simulink model "gm_DUALportRAMinterface_v3_vnl"  (R2024a)
settings: Solver=FixedStepDiscrete  StartTime=0.0  StopTime=20  RelTol=1e-3
undefined symbols (not defined in the file or in its folder): magnitude, Ts
libraries: hdlsllib x419, hdlmdlgenlib x103, embmathops x12, simulink x5, dsphdlxfrm2 x2
(part 4 of 11)

== system gm_DUALportRAMinterface_v3_vnl/PL/integration_block1/GA_main/Chart ==
  sort_done : Inport  OutDataTypeStr=boolean  PortDimensions=1  SampleTime=3.00000003e-08
  start_GA : Inport  Port=2  OutDataTypeStr=boolean  PortDimensions=1  SampleTime=3.00000003e-08
  score_done : Inport  Port=3  OutDataTypeStr=boolean  PortDimensions=1  SampleTime=3.00000003e-08
  FIFO_full : Inport  Port=4  OutDataTypeStr=boolean  PortDimensions=1  SampleTime=3.00000003e-08
  random_gene : Inport  Port=5  OutDataTypeStr=fixdt(0, 3, 0)  PortDimensions=1  SampleTime=3.00000003e-08
  selected_method : Inport  Port=6  OutDataTypeStr=fixdt(0, 3, 0)  PortDimensions=1  SampleTime=3.00000003e-08
  sample_index : Inport  Port=7  OutDataTypeStr=fixdt(0, 4, 0)  PortDimensions=1  SampleTime=3.00000003e-08
  generation_counter : Inport  Port=8  OutDataTypeStr=uint16  PortDimensions=1  SampleTime=3.00000003e-08
  Chart : Stateflow chart  TreatAsAtomicUnit=on
      settings: PortSchema="{\"entries\":[{\"content\":{\"sides\":[{\"content\":{\"connectorIds\":[\"In1\",\"In2\",\"In3\",\"In4\",\"In5\",\"In6\",\"In7\",\"In8\"]},\"type\":\"ConnectorPlacement.EquallySpacedRectSide\",\"uuid\":\"62d80992-ebbf-487b-a33b-520d46b16df9\"},{\"content\":{\"connectorIds\":[\"Out1\",\"Out4\",\"Out5\",\"Out6\",\"Out8\",\"Out9\",\"Out7\",\"Out10\",\"Out11\",\"Out12\",\"Out15\",\"Out16\",\"Out13\",\"Out14\",\"Out3\",\"Out2\",\"Out17\",\"Out18\"],\"side\":\"RIGHT\"},\"type\":\"ConnectorPlacement.EquallySpacedRectSide\",\"uuid\":\"bfd840c0-5c4c-4a80-a2e3-fe311b40edf5\"},{\"content\":{\"side\":\"TOP\"},\"type\":\"ConnectorPlacement.EquallySpacedRectSide\",\"uuid\":\"4ac6e66e-dbf9-46cb-9f74-339923e0521f\"},{\"content\":{\"side\":\"BOTTOM\"},\"type\":\"ConnectorPlacement.EquallySpacedRectSide\",\"uuid\":\"c9defcd3-49e4-4e79-8497-0d4d1ccc3a89\"}]},\"type\":\"ConnectorPlacement.EquallySpacedConnector\",\"uuid\":\"f0f6ce29-0824-409a-b95e-7d534cdcf216\"}],\"packageUris\":[\"http://schema.mathworks.com/mf0/Connector/R2020b\"],\"version\":\"1.0\"}"
  GA_done : Outport  SampleTime=3.00000003e-08
  index_reset : Outport  Port=2  SampleTime=3.00000003e-08
  index_increment : Outport  Port=3  SampleTime=3.00000003e-08
  a2_method : Outport  Port=4  SampleTime=3.00000003e-08
  a3_method : Outport  Port=5  SampleTime=3.00000003e-08
  a4_method : Outport  Port=6  SampleTime=3.00000003e-08
  b4_method : Outport  Port=7  SampleTime=3.00000003e-08
  b2_method : Outport  Port=8  SampleTime=3.00000003e-08
  b3_method : Outport  Port=9  SampleTime=3.00000003e-08
  slave_input : Outport  Port=10  SampleTime=3.00000003e-08
  slave_output : Outport  Port=11  SampleTime=3.00000003e-08
  master_input : Outport  Port=12  SampleTime=3.00000003e-08
  generation_increment : Outport  Port=13  SampleTime=3.00000003e-08
  generation_reset : Outport  Port=14  SampleTime=3.00000003e-08
  master_output : Outport  Port=15  SampleTime=3.00000003e-08
  master_sort : Outport  Port=16  SampleTime=3.00000003e-08
  FIFO_out_en : Outport  Port=17  SampleTime=3.00000003e-08
  load_fifo : Outport  Port=18  SampleTime=3.00000003e-08
  wires:
  Chart/18(load_fifo) -> load_fifo/1
  Chart/17(FIFO_out_en) -> FIFO_out_en/1
  Chart/16(master_sort) -> master_sort/1
  Chart/15(master_output) -> master_output/1
  Chart/14(generation_reset) -> generation_reset/1
  Chart/13(generation_increment) -> generation_increment/1
  Chart/12(master_input) -> master_input/1
  Chart/11(slave_output) -> slave_output/1
  Chart/10(slave_input) -> slave_input/1
  Chart/9(b3_method) -> b3_method/1
  Chart/8(b2_method) -> b2_method/1
  Chart/7(b4_method) -> b4_method/1
  Chart/6(a4_method) -> a4_method/1
  Chart/5(a3_method) -> a3_method/1
  Chart/4(a2_method) -> a2_method/1
  Chart/3(index_increment) -> index_increment/1
  Chart/2(index_reset) -> index_reset/1
  Chart/1(GA_done) -> GA_done/1
  generation_counter/1 -> Chart/8(generation_counter)
  sample_index/1 -> Chart/7(sample_index)
  selected_method/1 -> Chart/6(selected_method)
  random_gene/1 -> Chart/5(random_gene)
  FIFO_full/1 -> Chart/4(FIFO_full)
  score_done/1 -> Chart/3(score_done)
  start_GA/1 -> Chart/2(start_GA)
  sort_done/1 -> Chart/1(sort_done)

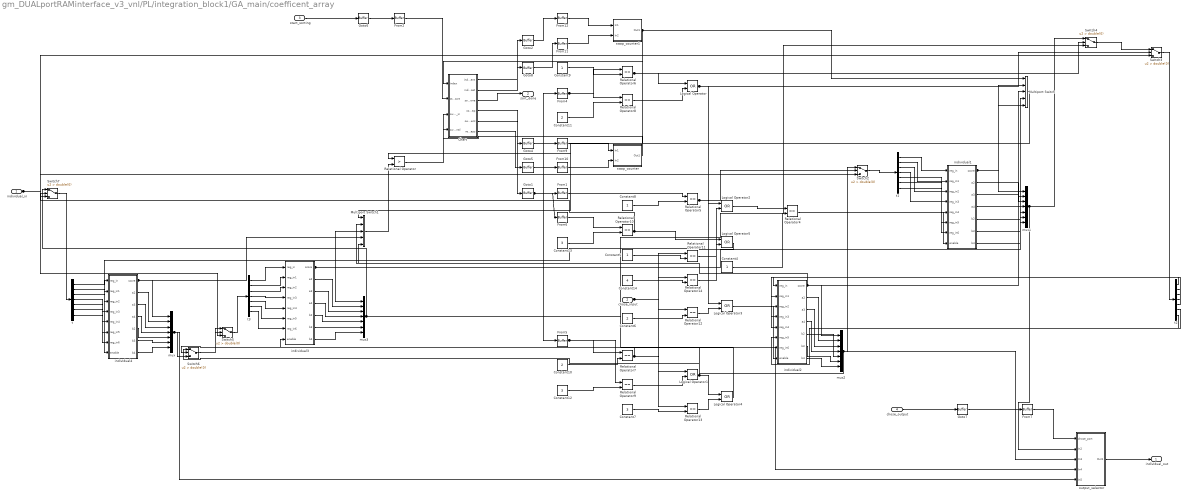
== system gm_DUALportRAMinterface_v3_vnl/PL/integration_block1/GA_main/coefficent_array ==
  individual_in : Inport  OutDataTypeStr=fixdt(1, 33, 15)  PortDimensions=[7]  SampleTime=3.00000003e-08
  chose_input : Inport  Port=2  OutDataTypeStr=fixdt(0, 4, 0)  PortDimensions=1  SampleTime=3.00000003e-08
  start_sorting : Inport  Port=3  OutDataTypeStr=boolean  PortDimensions=1  SampleTime=3.00000003e-08
  chose_output : Inport  Port=4  OutDataTypeStr=fixdt(0, 4, 0)  PortDimensions=1  SampleTime=3.00000003e-08
  Chart : Subsystem
  Constant10 : Constant  Value=2  OutDataTypeStr=fixdt(0, 4, 0)  SampleTime=3.00000003e-08
  Constant11 : Constant  Value=2  OutDataTypeStr=fixdt(0, 4, 0)  SampleTime=3.00000003e-08
  Constant12 : Constant  Value=3  OutDataTypeStr=fixdt(0, 4, 0)  SampleTime=3.00000003e-08
  Constant13 : Constant  Value=3  OutDataTypeStr=fixdt(0, 4, 0)  SampleTime=3.00000003e-08
  Constant14 : Constant  Value=4  OutDataTypeStr=fixdt(0, 4, 0)  SampleTime=3.00000003e-08
  Constant{4..5,8..9} (4 alike) : Constant  OutDataTypeStr=fixdt(0, 4, 0)  SampleTime=3.00000003e-08
  Constant6 : Constant  Value=2  OutDataTypeStr=fixdt(0, 4, 0)  SampleTime=3.00000003e-08
  Constant7 : Constant  Value=3  OutDataTypeStr=fixdt(0, 4, 0)  SampleTime=3.00000003e-08
  From{1..2,4..7,9..12} (10 alike) : hdlmdlgenlib/Buffer
  Goto{1..2,4..8} (7 alike) : hdlmdlgenlib/Buffer
  Logical Operator{,1..5} (6 alike) : Logic  Operator=OR  AllPortsSameDT=off  OutDataTypeStr=boolean  SampleTime=3.00000003e-08
  Multiport Switch : MultiPortSwitch  DataPortForDefault=Additional data port  DiagnosticForDefault=None  OutDataTypeStr=fixdt(1, 33, 15)  SampleTime=3.00000003e-08  SaturateOnIntegerOverflow=off  InputSameDT=off
  Multiport Switch1 : MultiPortSwitch  DataPortForDefault=Additional data port  DiagnosticForDefault=None  OutDataTypeStr=fixdt(1, 33, 15)  SampleTime=3.00000003e-08  SaturateOnIntegerOverflow=off  InputSameDT=off
  Relational Operator : RelationalOperator  Operator=>  OutDataTypeStr=boolean  SampleTime=3.00000003e-08  InputSameDT=off
  Relational Operator{4..14} (11 alike) : RelationalOperator  Operator===  OutDataTypeStr=boolean  SampleTime=3.00000003e-08  InputSameDT=off
  Switch{2..7} (6 alike) : Switch  Criteria=u2 > Threshold  Threshold=double(0)  OutDataTypeStr=fixdt(1, 33, 15)  SampleTime=3.00000003e-08  SaturateOnIntegerOverflow=off  InputSameDT=off
  individual1 : Subsystem
  individual2 : Subsystem
  individual3 : Subsystem
  individual4 : Subsystem
  mux{,1..3} (4 alike) : Mux  Inputs=7
  output_selector : Subsystem
  swap_counter : Subsystem
  swap_counter1 : Subsystem
  t{,1..3} (4 alike) : Demux  Outputs=7
  individual_out : Outport  SampleTime=3.00000003e-08
  sort_done : Outport  Port=2  SampleTime=3.00000003e-08
  wires:
  Switch5/1 -> t3/1
  Switch6/1 -> Switch5/1
  Switch3/1 -> t2/1
  Switch4/1 -> Switch3/1
  Switch2/1 -> t1/1
  Relational Operator5/1 -> Logical Operator2/1, Switch2/2
  From1/1 -> Relational Operator5/1
  Goto1/1 -> From1/1, From4/1, From5/1, From6/1
  Chart/6(reset_swaps) -> Goto5/1
  Chart/5(swaps_increment) -> Goto4/1
  Chart/4(commit_swap) -> Goto1/1
  Chart/2(index_reset) -> Goto8/1
  Chart/1(index_increment) -> Goto2/1
  Goto2/1 -> From12/1
  Goto8/1 -> From11/1
  Goto4/1 -> From9/1
  Goto5/1 -> From10/1
  Relational Operator/1 -> Chart/4(swap_signal)
  Multiport Switch/1 -> Relational Operator/1
  Multiport Switch1/1 -> Relational Operator/2
  Switch7/1 -> t/1
  Relational Operator10/1 -> Logical Operator5/1, Switch7/2
  From6/1 -> Relational Operator10/1
  Logical Operator2/1 -> Relational Operator4/1
  Relational Operator6/1 -> Logical Operator/1, Switch4/2
  From4/1 -> Relational Operator6/1, Relational Operator8/1
  Logical Operator/1 -> Logical Operator3/1, Switch3/2
  Relational Operator8/1 -> Logical Operator/2
  Relational Operator7/1 -> Logical Operator1/1, Switch6/2
  From5/1 -> Relational Operator7/1, Relational Operator9/1
  Logical Operator1/1 -> Logical Operator4/1, Switch5/2
  Relational Operator9/1 -> Logical Operator1/2
  t3/7 -> individual3/7(reg_in6)
  t3/6 -> individual3/6(reg_in5)
  t3/5 -> individual3/5(reg_in4)
  t3/4 -> individual3/4(reg_in3)
  t3/3 -> individual3/3(reg_in2)
  t3/2 -> individual3/2(reg_in1)
  t3/1 -> individual3/1(reg_in)
  t2/7 -> individual2/7(reg_in6)
  t2/6 -> individual2/6(reg_in5)
  t2/5 -> individual2/5(reg_in4)
  t2/4 -> individual2/4(reg_in3)
  t2/3 -> individual2/3(reg_in2)
  t2/2 -> individual2/2(reg_in1)
  t2/1 -> individual2/1(reg_in)
  t1/7 -> individual1/7(reg_in6)
  t1/6 -> individual1/6(reg_in5)
  t1/5 -> individual1/5(reg_in4)
  t1/4 -> individual1/4(reg_in3)
  t1/3 -> individual1/3(reg_in2)
  t1/2 -> individual1/2(reg_in1)
  t1/1 -> individual1/1(reg_in)
  From12/1 -> swap_counter1/1(In1)
  From11/1 -> swap_counter1/2(In2)
  From9/1 -> swap_counter/1(In1)
  From10/1 -> swap_counter/2(In2)
  t/7 -> individual4/7(reg_in6)
  t/6 -> individual4/6(reg_in5)
  t/5 -> individual4/5(reg_in4)
  t/4 -> individual4/4(reg_in3)
  t/3 -> individual4/3(reg_in2)
  t/2 -> individual4/2(reg_in1)
  t/1 -> individual4/1(reg_in)
  Logical Operator5/1 -> individual4/8(enable)
  Relational Operator4/1 -> individual1/8(enable)
  Logical Operator3/1 -> individual2/8(enable)
  Logical Operator4/1 -> individual3/8(enable)
  Constant8/1 -> Relational Operator5/2
  From2/1 -> Chart/2(start_sort)
  individual_in/1 -> Switch2/3, Switch3/3, Switch5/3, Switch7/3
  Constant13/1 -> Relational Operator10/2
  Relational Operator14/1 -> Logical Operator5/2
  Constant4/1 -> Relational Operator4/2
  Relational Operator11/1 -> Logical Operator2/2
  Constant9/1 -> Relational Operator6/2
  Constant11/1 -> Relational Operator8/2
  Relational Operator12/1 -> Logical Operator3/2
  Constant10/1 -> Relational Operator7/2
  Constant12/1 -> Relational Operator9/2
  Relational Operator13/1 -> Logical Operator4/2
  swap_counter1/1(Out1) -> Multiport Switch1/1, Multiport Switch/1, Chart/1(index)
  swap_counter/1(Out1) -> Chart/3(swaps_in)
  individual4/7(b4) -> mux/7
  individual4/6(b3) -> mux/6
  individual4/5(b2) -> mux/5
  individual4/4(a4) -> mux/4
  individual4/3(a3) -> mux/3
  individual4/2(a2) -> mux/2
  individual4/1(score) -> mux/1, Multiport Switch1/4
  individual1/7(b4) -> mux1/7
  individual1/6(b3) -> mux1/6
  individual1/5(b2) -> mux1/5
  individual1/4(a4) -> mux1/4
  individual1/3(a3) -> mux1/3
  individual1/2(a2) -> mux1/2
  individual1/1(score) -> mux1/1, Multiport Switch/5, Multiport Switch/2
  individual2/7(b4) -> mux2/7
  individual2/6(b3) -> mux2/6
  individual2/5(b2) -> mux2/5
  individual2/4(a4) -> mux2/4
  individual2/3(a3) -> mux2/3
  individual2/2(a2) -> mux2/2
  individual2/1(score) -> mux2/1, Multiport Switch1/5, Multiport Switch1/2, Multiport Switch/3
  individual3/7(b4) -> mux3/7
  individual3/6(b3) -> mux3/6
  individual3/5(b2) -> mux3/5
  individual3/4(a4) -> mux3/4
  individual3/3(a3) -> mux3/3
  individual3/2(a2) -> mux3/2
  individual3/1(score) -> mux3/1, Multiport Switch1/3, Multiport Switch/4
  Goto7/1 -> From7/1
  Goto6/1 -> From2/1
  output_selector/1(Out1) -> individual_out/1
  mux/1 -> Switch6/3, output_selector/5(In5)
  mux3/1 -> Switch4/3, Switch7/1, output_selector/4(In4)
  mux2/1 -> Switch2/1, Switch6/1, output_selector/3(In3)
  mux1/1 -> Switch4/1, output_selector/2(In2)
  From7/1 -> output_selector/1(chose_port)
  Constant7/1 -> Relational Operator13/2
  Constant6/1 -> Relational Operator12/2
  Constant5/1 -> Relational Operator11/2
  Constant14/1 -> Relational Operator14/2
  Chart/3(sort_done) -> sort_done/1
  chose_output/1 -> Goto7/1
  start_sorting/1 -> Goto6/1
  chose_input/1 -> Relational Operator11/1, Relational Operator12/1, Relational Operator13/1, Relational Operator14/1

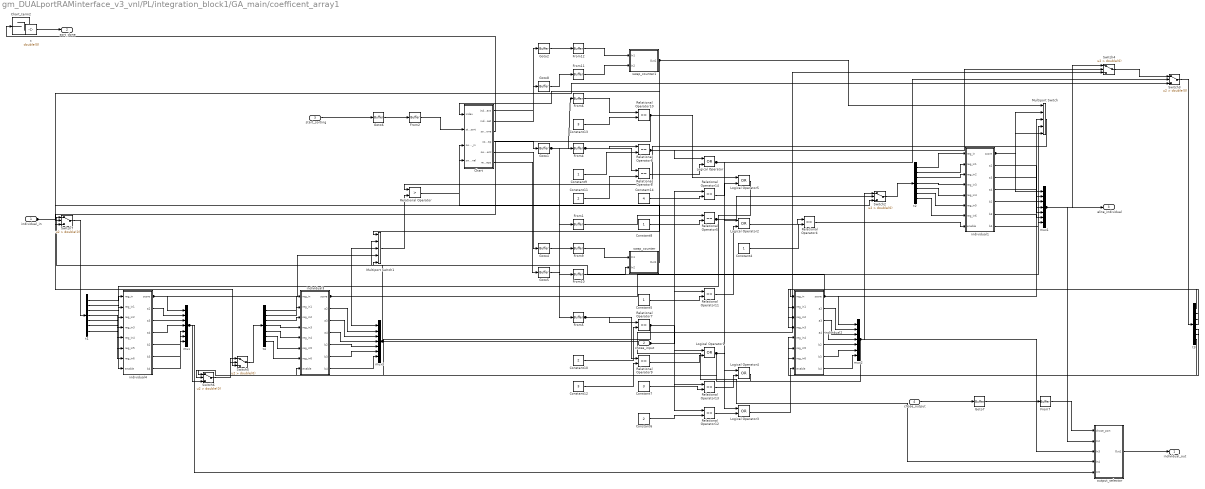
== system gm_DUALportRAMinterface_v3_vnl/PL/integration_block1/GA_main/coefficent_array1 ==
  individual_in : Inport  OutDataTypeStr=fixdt(1, 33, 15)  PortDimensions=[7]  SampleTime=3.00000003e-08
  chose_input : Inport  Port=2  OutDataTypeStr=fixdt(0, 4, 0)  PortDimensions=1  SampleTime=3.00000003e-08
  start_sorting : Inport  Port=3  OutDataTypeStr=boolean  PortDimensions=1  SampleTime=3.00000003e-08
  chose_output : Inport  Port=4  OutDataTypeStr=fixdt(0, 4, 0)  PortDimensions=1  SampleTime=3.00000003e-08
  Chart : Subsystem
  Chart_term2 : Terminator
  Constant10 : Constant  Value=2  OutDataTypeStr=fixdt(0, 4, 0)  SampleTime=3.00000003e-08
  Constant11 : Constant  Value=2  OutDataTypeStr=fixdt(0, 4, 0)  SampleTime=3.00000003e-08
  Constant12 : Constant  Value=3  OutDataTypeStr=fixdt(0, 4, 0)  SampleTime=3.00000003e-08
  Constant13 : Constant  Value=3  OutDataTypeStr=fixdt(0, 4, 0)  SampleTime=3.00000003e-08
  Constant14 : Constant  Value=4  OutDataTypeStr=fixdt(0, 4, 0)  SampleTime=3.00000003e-08
  Constant{4..5,8..9} (4 alike) : Constant  OutDataTypeStr=fixdt(0, 4, 0)  SampleTime=3.00000003e-08
  Constant6 : Constant  Value=2  OutDataTypeStr=fixdt(0, 4, 0)  SampleTime=3.00000003e-08
  Constant7 : Constant  Value=3  OutDataTypeStr=fixdt(0, 4, 0)  SampleTime=3.00000003e-08
  From{1..2,4..7,9..12} (10 alike) : hdlmdlgenlib/Buffer
  Goto{1..2,4..8} (7 alike) : hdlmdlgenlib/Buffer
  Logical Operator{,1..5} (6 alike) : Logic  Operator=OR  AllPortsSameDT=off  OutDataTypeStr=boolean  SampleTime=3.00000003e-08
  Multiport Switch : MultiPortSwitch  DataPortForDefault=Additional data port  DiagnosticForDefault=None  OutDataTypeStr=fixdt(1, 33, 15)  SampleTime=3.00000003e-08  SaturateOnIntegerOverflow=off  InputSameDT=off
  Multiport Switch1 : MultiPortSwitch  DataPortForDefault=Additional data port  DiagnosticForDefault=None  OutDataTypeStr=fixdt(1, 33, 15)  SampleTime=3.00000003e-08  SaturateOnIntegerOverflow=off  InputSameDT=off
  Relational Operator : RelationalOperator  Operator=>  OutDataTypeStr=boolean  SampleTime=3.00000003e-08  InputSameDT=off
  Relational Operator{4..14} (11 alike) : RelationalOperator  Operator===  OutDataTypeStr=boolean  SampleTime=3.00000003e-08  InputSameDT=off
  Switch{2..7} (6 alike) : Switch  Criteria=u2 > Threshold  Threshold=double(0)  OutDataTypeStr=fixdt(1, 33, 15)  SampleTime=3.00000003e-08  SaturateOnIntegerOverflow=off  InputSameDT=off
  individual1 : Subsystem
  individual2 : Subsystem
  individual3 : Subsystem
  individual4 : Subsystem
  mux{,1..3} (4 alike) : Mux  Inputs=7
  output_selector : Subsystem
  swap_counter : Subsystem
  swap_counter1 : Subsystem
  t : Constant  Value=double(0)  OutDataTypeStr=boolean  SampleTime=3.00000003e-08
  t{1..4} (4 alike) : Demux  Outputs=7
  individual_out : Outport  SampleTime=3.00000003e-08
  sort_done : Outport  Port=2  SampleTime=3.00000003e-08
  elite_individual : Outport  Port=3  SampleTime=3.00000003e-08
  wires:
  Switch5/1 -> t4/1
  Switch6/1 -> Switch5/1
  Switch3/1 -> t3/1
  Switch4/1 -> Switch3/1
  Switch2/1 -> t2/1
  Relational Operator5/1 -> Logical Operator2/1, Switch2/2
  From1/1 -> Relational Operator5/1
  Goto1/1 -> From1/1, From4/1, From5/1, From6/1
  Chart/6(reset_swaps) -> Goto5/1
  Chart/5(swaps_increment) -> Goto4/1
  Chart/4(commit_swap) -> Goto1/1
  Chart/2(index_reset) -> Goto8/1
  Chart/1(index_increment) -> Goto2/1
  Goto2/1 -> From12/1
  Goto8/1 -> From11/1
  Goto4/1 -> From9/1
  Goto5/1 -> From10/1
  Relational Operator/1 -> Chart/4(swap_signal)
  Multiport Switch/1 -> Relational Operator/1
  Multiport Switch1/1 -> Relational Operator/2
  Switch7/1 -> t1/1
  Relational Operator10/1 -> Logical Operator5/1, Switch7/2
  From6/1 -> Relational Operator10/1
  Logical Operator2/1 -> Relational Operator4/1
  Relational Operator6/1 -> Logical Operator/1, Switch4/2
  From4/1 -> Relational Operator6/1, Relational Operator8/1
  Logical Operator/1 -> Logical Operator3/1, Switch3/2
  Relational Operator8/1 -> Logical Operator/2
  Relational Operator7/1 -> Logical Operator1/1, Switch6/2
  From5/1 -> Relational Operator7/1, Relational Operator9/1
  Logical Operator1/1 -> Logical Operator4/1, Switch5/2
  Relational Operator9/1 -> Logical Operator1/2
  t4/7 -> individual3/7(reg_in6)
  t4/6 -> individual3/6(reg_in5)
  t4/5 -> individual3/5(reg_in4)
  t4/4 -> individual3/4(reg_in3)
  t4/3 -> individual3/3(reg_in2)
  t4/2 -> individual3/2(reg_in1)
  t4/1 -> individual3/1(reg_in)
  t3/7 -> individual2/7(reg_in6)
  t3/6 -> individual2/6(reg_in5)
  t3/5 -> individual2/5(reg_in4)
  t3/4 -> individual2/4(reg_in3)
  t3/3 -> individual2/3(reg_in2)
  t3/2 -> individual2/2(reg_in1)
  t3/1 -> individual2/1(reg_in)
  t2/7 -> individual1/7(reg_in6)
  t2/6 -> individual1/6(reg_in5)
  t2/5 -> individual1/5(reg_in4)
  t2/4 -> individual1/4(reg_in3)
  t2/3 -> individual1/3(reg_in2)
  t2/2 -> individual1/2(reg_in1)
  t2/1 -> individual1/1(reg_in)
  From12/1 -> swap_counter1/1(In1)
  From11/1 -> swap_counter1/2(In2)
  From9/1 -> swap_counter/1(In1)
  From10/1 -> swap_counter/2(In2)
  t1/7 -> individual4/7(reg_in6)
  t1/6 -> individual4/6(reg_in5)
  t1/5 -> individual4/5(reg_in4)
  t1/4 -> individual4/4(reg_in3)
  t1/3 -> individual4/3(reg_in2)
  t1/2 -> individual4/2(reg_in1)
  t1/1 -> individual4/1(reg_in)
  Logical Operator5/1 -> individual4/8(enable)
  Relational Operator4/1 -> individual1/8(enable)
  Logical Operator3/1 -> individual2/8(enable)
  Logical Operator4/1 -> individual3/8(enable)
  Constant8/1 -> Relational Operator5/2
  From2/1 -> Chart/2(start_sort)
  individual_in/1 -> Switch2/3, Switch3/3, Switch5/3, Switch7/3
  Constant13/1 -> Relational Operator10/2
  Relational Operator14/1 -> Logical Operator5/2
  Constant4/1 -> Relational Operator4/2
  Relational Operator11/1 -> Logical Operator2/2
  Constant9/1 -> Relational Operator6/2
  Constant11/1 -> Relational Operator8/2
  Relational Operator12/1 -> Logical Operator3/2
  Constant10/1 -> Relational Operator7/2
  Constant12/1 -> Relational Operator9/2
  Relational Operator13/1 -> Logical Operator4/2
  swap_counter1/1(Out1) -> Multiport Switch1/1, Multiport Switch/1, Chart/1(index)
  swap_counter/1(Out1) -> Chart/3(swaps_in)
  individual4/7(b4) -> mux/7
  individual4/6(b3) -> mux/6
  individual4/5(b2) -> mux/5
  individual4/4(a4) -> mux/4
  individual4/3(a3) -> mux/3
  individual4/2(a2) -> mux/2
  individual4/1(score) -> mux/1, Multiport Switch1/4
  individual1/7(b4) -> mux1/7
  individual1/6(b3) -> mux1/6
  individual1/5(b2) -> mux1/5
  individual1/4(a4) -> mux1/4
  individual1/3(a3) -> mux1/3
  individual1/2(a2) -> mux1/2
  individual1/1(score) -> mux1/1, Multiport Switch/5, Multiport Switch/2
  individual2/7(b4) -> mux2/7
  individual2/6(b3) -> mux2/6
  individual2/5(b2) -> mux2/5
  individual2/4(a4) -> mux2/4
  individual2/3(a3) -> mux2/3
  individual2/2(a2) -> mux2/2
  individual2/1(score) -> mux2/1, Multiport Switch1/5, Multiport Switch1/2, Multiport Switch/3
  individual3/7(b4) -> mux3/7
  individual3/6(b3) -> mux3/6
  individual3/5(b2) -> mux3/5
  individual3/4(a4) -> mux3/4
  individual3/3(a3) -> mux3/3
  individual3/2(a2) -> mux3/2
  individual3/1(score) -> mux3/1, Multiport Switch1/3, Multiport Switch/4
  Chart/3(sort_done) -> Chart_term2/1
  Goto7/1 -> From7/1
  Goto6/1 -> From2/1
  output_selector/1(Out1) -> individual_out/1
  mux/1 -> Switch6/3, output_selector/5(In5)
  mux3/1 -> Switch4/3, Switch7/1, output_selector/4(In4)
  mux2/1 -> Switch2/1, Switch6/1, output_selector/3(In3)
  mux1/1 -> Switch4/1, output_selector/2(In2), elite_individual/1
  From7/1 -> output_selector/1(chose_port)
  Constant7/1 -> Relational Operator13/2
  Constant6/1 -> Relational Operator12/2
  Constant5/1 -> Relational Operator11/2
  Constant14/1 -> Relational Operator14/2
  t/1 -> sort_done/1
  chose_output/1 -> Goto7/1
  start_sorting/1 -> Goto6/1
  chose_input/1 -> Relational Operator11/1, Relational Operator12/1, Relational Operator13/1, Relational Operator14/1

== system gm_DUALportRAMinterface_v3_vnl/PL/integration_block1/GA_main/generation_counter ==
  In1 : Inport  OutDataTypeStr=boolean  PortDimensions=1  SampleTime=3.00000003e-08
  In2 : Inport  Port=2  OutDataTypeStr=boolean  PortDimensions=1  SampleTime=3.00000003e-08
  Add : Sum  OutDataTypeStr=fixdt(0,16,0)  AccumDataTypeStr=fixdt(0,16,0)
  Constant18 : Constant  OutDataTypeStr=fixdt(0,16,0)  SampleTime=Ts
  Constant19 : Constant  Value=0  OutDataTypeStr=fixdt(0,16,0)  SampleTime=Ts
  Constant20 : Constant  Value=0  OutDataTypeStr=fixdt(0,16,0)  SampleTime=Ts
  Delay : Delay  DelayLength=1  InitialCondition=0  SampleTime=Ts
  Switch : Switch  Criteria=u2 > Threshold  OutDataTypeStr=fixdt(0,16,0)  SaturateOnIntegerOverflow=off  InputSameDT=off
  Switch8 : Switch  Criteria=u2 > Threshold  OutDataTypeStr=fixdt(0,16,0)  SaturateOnIntegerOverflow=off  InputSameDT=off
  Out1 : Outport  SampleTime=3.00000003e-08
  wires:
  Switch8/1 -> Add/2
  Add/1 -> Delay/1
  Switch/1 -> Add/1
  In2/1 -> Switch8/2
  Constant20/1 -> Switch8/1
  Delay/1 -> Switch8/3, Out1/1
  Constant19/1 -> Switch/3
  Constant18/1 -> Switch/1
  In1/1 -> Switch/2

== system gm_DUALportRAMinterface_v3_vnl/PL/integration_block1/GA_main/index_counter ==
  In1 : Inport  OutDataTypeStr=boolean  PortDimensions=1  SampleTime=3.00000003e-08
  In2 : Inport  Port=2  OutDataTypeStr=boolean  PortDimensions=1  SampleTime=3.00000003e-08
  Add : Sum  OutDataTypeStr=fixdt(0,4,0)  AccumDataTypeStr=fixdt(0,4,0)
  Constant18 : Constant  OutDataTypeStr=fixdt(0,4,0)  SampleTime=Ts
  Constant19 : Constant  Value=0  OutDataTypeStr=fixdt(0,4,0)  SampleTime=Ts
  Constant20 : Constant  Value=0  OutDataTypeStr=fixdt(0,4,0)  SampleTime=Ts
  Delay : Delay  DelayLength=1  InitialCondition=0  SampleTime=Ts
  Switch : Switch  Criteria=u2 > Threshold  OutDataTypeStr=fixdt(0,4,0)  SaturateOnIntegerOverflow=off  InputSameDT=off
  Switch8 : Switch  Criteria=u2 > Threshold  OutDataTypeStr=fixdt(0,4,0)  SaturateOnIntegerOverflow=off  InputSameDT=off
  index_counter : Outport  SampleTime=3.00000003e-08
  wires:
  Switch8/1 -> Add/2
  Add/1 -> Delay/1
  Switch/1 -> Add/1
  In2/1 -> Switch8/2
  Constant20/1 -> Switch8/1
  Delay/1 -> Switch8/3, index_counter/1
  Constant19/1 -> Switch/3
  Constant18/1 -> Switch/1
  In1/1 -> Switch/2

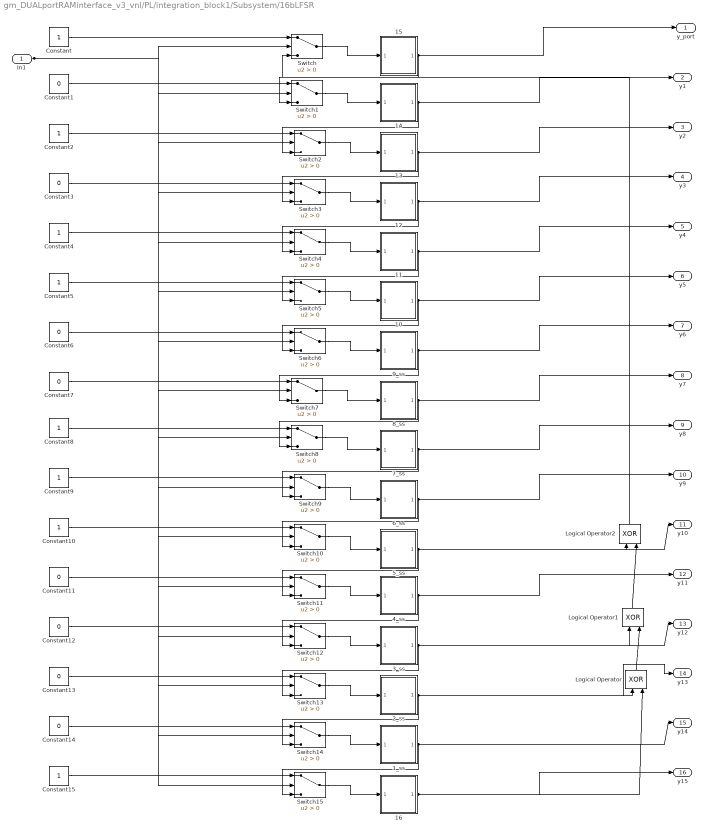
== system gm_DUALportRAMinterface_v3_vnl/PL/integration_block1/Subsystem/16bLFSR ==
  In1 : Inport  OutDataTypeStr=boolean  PortDimensions=1  SampleTime=3.00000003e-08
  10 : Subsystem
  11 : Subsystem
  12 : Subsystem
  13 : Subsystem
  14 : Subsystem
  15 : Subsystem
  16 : Subsystem
  1_ss : Subsystem
  2_ss : Subsystem
  3_ss : Subsystem
  4_ss : Subsystem
  5_ss : Subsystem
  6_ss : Subsystem
  7_ss : Subsystem
  8_ss : Subsystem
  9_ss : Subsystem
  Constant{,2,4..5,8..10,15} (8 alike) : Constant  OutDataTypeStr=boolean  SampleTime=Ts
  Constant{1,3,6..7,11..14} (8 alike) : Constant  Value=0  OutDataTypeStr=boolean  SampleTime=Ts
  Logical Operator : Logic  Operator=XOR  IconShape=distinctive  AllPortsSameDT=off  OutDataTypeStr=boolean
  Logical Operator1 : Logic  Operator=XOR  IconShape=distinctive  AllPortsSameDT=off  OutDataTypeStr=boolean
  Logical Operator2 : Logic  Operator=XOR  IconShape=distinctive  AllPortsSameDT=off  OutDataTypeStr=boolean
  Switch{,1..15} (16 alike) : Switch  Criteria=u2 > Threshold  OutDataTypeStr=boolean  SaturateOnIntegerOverflow=off  InputSameDT=off
  y_port : Outport  SampleTime=3.00000003e-08
  y1 : Outport  Port=2  SampleTime=3.00000003e-08
  y2 : Outport  Port=3  SampleTime=3.00000003e-08
  y3 : Outport  Port=4  SampleTime=3.00000003e-08
  y4 : Outport  Port=5  SampleTime=3.00000003e-08
  y5 : Outport  Port=6  SampleTime=3.00000003e-08
  y6 : Outport  Port=7  SampleTime=3.00000003e-08
  y7 : Outport  Port=8  SampleTime=3.00000003e-08
  y8 : Outport  Port=9  SampleTime=3.00000003e-08
  y9 : Outport  Port=10  SampleTime=3.00000003e-08
  y10 : Outport  Port=11  SampleTime=3.00000003e-08
  y11 : Outport  Port=12  SampleTime=3.00000003e-08
  y12 : Outport  Port=13  SampleTime=3.00000003e-08
  y13 : Outport  Port=14  SampleTime=3.00000003e-08
  y14 : Outport  Port=15  SampleTime=3.00000003e-08
  y15 : Outport  Port=16  SampleTime=3.00000003e-08
  wires:
  Switch14/1 -> 1_ss/1(reg_in)
  Switch13/1 -> 2_ss/1(reg_in)
  Switch12/1 -> 3_ss/1(reg_in)
  Switch11/1 -> 4_ss/1(reg_in)
  Switch10/1 -> 5_ss/1(reg_in)
  Switch9/1 -> 6_ss/1(reg_in)
  Switch8/1 -> 7_ss/1(reg_in)
  Switch7/1 -> 8_ss/1(reg_in)
  Switch6/1 -> 9_ss/1(reg_in)
  Switch5/1 -> 10/1(reg_in)
  Switch4/1 -> 11/1(reg_in)
  Switch3/1 -> 12/1(reg_in)
  Switch2/1 -> 13/1(reg_in)
  Switch1/1 -> 14/1(reg_in)
  Logical Operator2/1 -> Switch/3
  Logical Operator1/1 -> Logical Operator2/2
  Logical Operator/1 -> Logical Operator1/2
  Switch/1 -> 15/1(reg_in)
  Switch15/1 -> 16/1(reg_in)
  Constant14/1 -> Switch14/1
  Constant13/1 -> Switch13/1
  Constant12/1 -> Switch12/1
  Constant11/1 -> Switch11/1
  Constant10/1 -> Switch10/1
  Constant9/1 -> Switch9/1
  Constant8/1 -> Switch8/1
  Constant7/1 -> Switch7/1
  Constant6/1 -> Switch6/1
  Constant5/1 -> Switch5/1
  Constant4/1 -> Switch4/1
  Constant3/1 -> Switch3/1
  Constant2/1 -> Switch2/1
  Constant1/1 -> Switch1/1
  Constant/1 -> Switch/1
  Constant15/1 -> Switch15/1
  9_ss/1(reg_out) -> Switch7/3, y6/1
  8_ss/1(reg_out) -> Switch8/3, y7/1
  7_ss/1(reg_out) -> Switch9/3, y8/1
  6_ss/1(reg_out) -> Switch10/3, y9/1
  5_ss/1(reg_out) -> Logical Operator2/1, Switch11/3, y10/1
  4_ss/1(reg_out) -> Switch12/3, y11/1
  3_ss/1(reg_out) -> Logical Operator1/1, Switch13/3, y12/1
  2_ss/1(reg_out) -> Logical Operator/1, Switch14/3, y13/1
  1_ss/1(reg_out) -> Switch15/3, y14/1
  16/1(reg_out) -> Logical Operator/2, y15/1
  15/1(reg_out) -> Switch1/3, y_port/1
  14/1(reg_out) -> Switch2/3, y1/1
  13/1(reg_out) -> Switch3/3, y2/1
  12/1(reg_out) -> Switch4/3, y3/1
  11/1(reg_out) -> Switch5/3, y4/1
  10/1(reg_out) -> Switch6/3, y5/1
  In1/1 -> Switch14/2, Switch13/2, Switch12/2, Switch11/2, Switch10/2, Switch9/2, Switch8/2, Switch7/2, Switch6/2, Switch5/2, Switch4/2, Switch3/2, Switch2/2, Switch1/2, Switch/2, Switch15/2

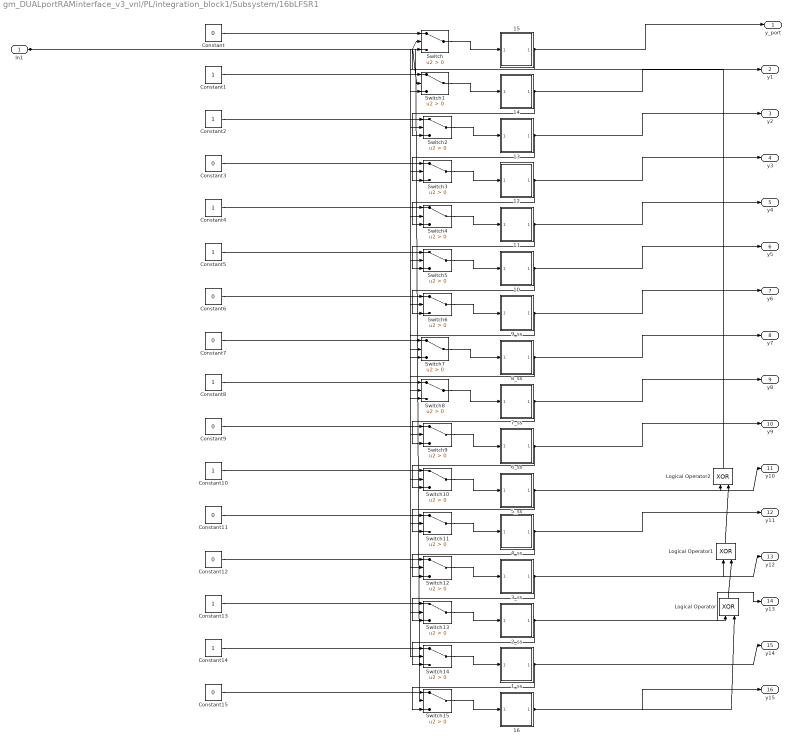
== system gm_DUALportRAMinterface_v3_vnl/PL/integration_block1/Subsystem/16bLFSR1 ==
  In1 : Inport  OutDataTypeStr=boolean  PortDimensions=1  SampleTime=3.00000003e-08
  10 : Subsystem
  11 : Subsystem
  12 : Subsystem
  13 : Subsystem
  14 : Subsystem
  15 : Subsystem
  16 : Subsystem
  1_ss : Subsystem
  2_ss : Subsystem
  3_ss : Subsystem
  4_ss : Subsystem
  5_ss : Subsystem
  6_ss : Subsystem
  7_ss : Subsystem
  8_ss : Subsystem
  9_ss : Subsystem
  Constant{,3,6..7,9,11..12,15} (8 alike) : Constant  Value=0  OutDataTypeStr=boolean  SampleTime=Ts
  Constant{1..2,4..5,8,10,13..14} (8 alike) : Constant  OutDataTypeStr=boolean  SampleTime=Ts
  Logical Operator : Logic  Operator=XOR  IconShape=distinctive  AllPortsSameDT=off  OutDataTypeStr=boolean
  Logical Operator1 : Logic  Operator=XOR  IconShape=distinctive  AllPortsSameDT=off  OutDataTypeStr=boolean
  Logical Operator2 : Logic  Operator=XOR  IconShape=distinctive  AllPortsSameDT=off  OutDataTypeStr=boolean
  Switch{,1..15} (16 alike) : Switch  Criteria=u2 > Threshold  OutDataTypeStr=boolean  SaturateOnIntegerOverflow=off  InputSameDT=off
  y_port : Outport  SampleTime=3.00000003e-08
  y1 : Outport  Port=2  SampleTime=3.00000003e-08
  y2 : Outport  Port=3  SampleTime=3.00000003e-08
  y3 : Outport  Port=4  SampleTime=3.00000003e-08
  y4 : Outport  Port=5  SampleTime=3.00000003e-08
  y5 : Outport  Port=6  SampleTime=3.00000003e-08
  y6 : Outport  Port=7  SampleTime=3.00000003e-08
  y7 : Outport  Port=8  SampleTime=3.00000003e-08
  y8 : Outport  Port=9  SampleTime=3.00000003e-08
  y9 : Outport  Port=10  SampleTime=3.00000003e-08
  y10 : Outport  Port=11  SampleTime=3.00000003e-08
  y11 : Outport  Port=12  SampleTime=3.00000003e-08
  y12 : Outport  Port=13  SampleTime=3.00000003e-08
  y13 : Outport  Port=14  SampleTime=3.00000003e-08
  y14 : Outport  Port=15  SampleTime=3.00000003e-08
  y15 : Outport  Port=16  SampleTime=3.00000003e-08
  wires:
  Switch14/1 -> 1_ss/1(reg_in)
  Switch13/1 -> 2_ss/1(reg_in)
  Switch12/1 -> 3_ss/1(reg_in)
  Switch11/1 -> 4_ss/1(reg_in)
  Switch10/1 -> 5_ss/1(reg_in)
  Switch9/1 -> 6_ss/1(reg_in)
  Switch8/1 -> 7_ss/1(reg_in)
  Switch7/1 -> 8_ss/1(reg_in)
  Switch6/1 -> 9_ss/1(reg_in)
  Switch5/1 -> 10/1(reg_in)
  Switch4/1 -> 11/1(reg_in)
  Switch3/1 -> 12/1(reg_in)
  Switch2/1 -> 13/1(reg_in)
  Switch1/1 -> 14/1(reg_in)
  Logical Operator2/1 -> Switch/3
  Logical Operator1/1 -> Logical Operator2/2
  Logical Operator/1 -> Logical Operator1/2
  Switch/1 -> 15/1(reg_in)
  Switch15/1 -> 16/1(reg_in)
  Constant14/1 -> Switch14/1
  Constant13/1 -> Switch13/1
  Constant12/1 -> Switch12/1
  Constant11/1 -> Switch11/1
  Constant10/1 -> Switch10/1
  Constant9/1 -> Switch9/1
  Constant8/1 -> Switch8/1
  Constant7/1 -> Switch7/1
  Constant6/1 -> Switch6/1
  Constant5/1 -> Switch5/1
  Constant4/1 -> Switch4/1
  Constant3/1 -> Switch3/1
  Constant2/1 -> Switch2/1
  Constant1/1 -> Switch1/1
  Constant/1 -> Switch/1
  Constant15/1 -> Switch15/1
  9_ss/1(reg_out) -> Switch7/3, y6/1
  8_ss/1(reg_out) -> Switch8/3, y7/1
  7_ss/1(reg_out) -> Switch9/3, y8/1
  6_ss/1(reg_out) -> Switch10/3, y9/1
  5_ss/1(reg_out) -> Logical Operator2/1, Switch11/3, y10/1
  4_ss/1(reg_out) -> Switch12/3, y11/1
  3_ss/1(reg_out) -> Logical Operator1/1, Switch13/3, y12/1
  2_ss/1(reg_out) -> Logical Operator/1, Switch14/3, y13/1
  1_ss/1(reg_out) -> Switch15/3, y14/1
  16/1(reg_out) -> Logical Operator/2, y15/1
  15/1(reg_out) -> Switch1/3, y_port/1
  14/1(reg_out) -> Switch2/3, y1/1
  13/1(reg_out) -> Switch3/3, y2/1
  12/1(reg_out) -> Switch4/3, y3/1
  11/1(reg_out) -> Switch5/3, y4/1
  10/1(reg_out) -> Switch6/3, y5/1
  In1/1 -> Switch14/2, Switch13/2, Switch12/2, Switch11/2, Switch10/2, Switch9/2, Switch8/2, Switch7/2, Switch6/2, Switch5/2, Switch4/2, Switch3/2, Switch2/2, Switch1/2, Switch/2, Switch15/2

== system gm_DUALportRAMinterface_v3_vnl/PL/integration_block1/Subsystem/a2_random ==
  In1 : Inport  OutDataTypeStr=uint16  PortDimensions=1  SampleTime=3.00000003e-08
  In2 : Inport  Port=2  OutDataTypeStr=boolean  PortDimensions=1  SampleTime=3.00000003e-08
  Add : Sum  Inputs=+-  OutDataTypeStr=fixdt(1, 18, 15)
  Add1 : Sum  OutDataTypeStr=fixdt(1, 17, 15)
  Bit Shift : hdlsllib/Logic and Bit Operations/Bit Shift  mode=Shift Right Logical  N=16+5
  Constant : Constant  OutDataTypeStr=boolean  SampleTime=Ts
  Constant16 : Constant  Value=-1.975  OutDataTypeStr=fixdt(1,18,15)  SampleTime=Ts
  Data Type Conversion : DataTypeConversion  OutDataTypeStr=fixdt(0,11,11)  SaturateOnIntegerOverflow=off  RndMeth=Floor
  Data Type Conversion1 : DataTypeConversion  OutDataTypeStr=fixdt(0,32,16)  SaturateOnIntegerOverflow=off  RndMeth=Floor
  Data Type Conversion2 : DataTypeConversion  OutDataTypeStr=fixdt(1,17,15)  SaturateOnIntegerOverflow=off  RndMeth=Floor
  Modulo by Constant HDL Optimized1 : embmathops/Modulo by Constant HDL Optimized  Denominator=0.025  SimulateUsing=Code generation
      settings: LibrarySourceBlock=|
      | embeddedMatrixLib/Math Operations/Modulo by Constant
      | HDL Optimized
  Switch16 : Switch  Criteria=u2 > Threshold  OutDataTypeStr=fixdt(1, 18, 15)  SaturateOnIntegerOverflow=off  InputSameDT=off
  mod_by_constant_term1 : Terminator
  Out1 : Outport  SampleTime=3.00000003e-08
  wires:
  Switch16/1 -> Out1/1
  Modulo by Constant HDL Optimized1/2 -> mod_by_constant_term1/1
  Modulo by Constant HDL Optimized1/1 -> Data Type Conversion2/1
  Data Type Conversion2/1 -> Add/2, Add1/1
  Data Type Conversion1/1 -> Bit Shift/1
  Data Type Conversion/1 -> Modulo by Constant HDL Optimized1/1
  Constant16/1 -> Add/1, Add1/2
  Constant/1 -> Modulo by Constant HDL Optimized1/2
  Bit Shift/1 -> Data Type Conversion/1
  Add1/1 -> Switch16/3
  Add/1 -> Switch16/1
  In2/1 -> Switch16/2
  In1/1 -> Data Type Conversion1/1

== system gm_DUALportRAMinterface_v3_vnl/PL/integration_block1/Subsystem/a3_random ==
  In1 : Inport  OutDataTypeStr=uint16  PortDimensions=1  SampleTime=3.00000003e-08
  In2 : Inport  Port=2  OutDataTypeStr=boolean  PortDimensions=1  SampleTime=3.00000003e-08
  Add6 : Sum  Inputs=+-  OutDataTypeStr=fixdt(1, 18, 15)
  Add7 : Sum  OutDataTypeStr=fixdt(1, 18, 15)
  Bit Shift3 : hdlsllib/Logic and Bit Operations/Bit Shift  mode=Shift Right Logical  N=16+6
  Constant : Constant  OutDataTypeStr=boolean  SampleTime=Ts
  Constant3 : Constant  Value=1.0286  OutDataTypeStr=fixdt(1,18,15)  SampleTime=Ts
  Data Type Conversion10 : DataTypeConversion  OutDataTypeStr=fixdt(0,32,16)  SaturateOnIntegerOverflow=off  RndMeth=Floor
  Data Type Conversion11 : DataTypeConversion  OutDataTypeStr=fixdt(1,18,15)  SaturateOnIntegerOverflow=off  RndMeth=Floor
  Data Type Conversion9 : DataTypeConversion  OutDataTypeStr=fixdt(0,11,11)  SaturateOnIntegerOverflow=off  RndMeth=Floor
  Modulo by Constant HDL Optimized : embmathops/Modulo by Constant HDL Optimized  Denominator=0.0106  SimulateUsing=Code generation
      settings: LibrarySourceBlock=|
      | embeddedMatrixLib/Math Operations/Modulo by Constant
      | HDL Optimized
  Switch3 : Switch  Criteria=u2 > Threshold  OutDataTypeStr=fixdt(1, 18, 15)  SaturateOnIntegerOverflow=off  InputSameDT=off
  mod_by_constant_term1 : Terminator
  Out1 : Outport  SampleTime=3.00000003e-08
  wires:
  Switch3/1 -> Out1/1
  Modulo by Constant HDL Optimized/2 -> mod_by_constant_term1/1
  Modulo by Constant HDL Optimized/1 -> Data Type Conversion11/1
  Data Type Conversion9/1 -> Modulo by Constant HDL Optimized/1
  Data Type Conversion11/1 -> Add6/2, Add7/1
  Data Type Conversion10/1 -> Bit Shift3/1
  Constant3/1 -> Add6/1, Add7/2
  Constant/1 -> Modulo by Constant HDL Optimized/2
  Bit Shift3/1 -> Data Type Conversion9/1
  Add7/1 -> Switch3/3
  Add6/1 -> Switch3/1
  In2/1 -> Switch3/2
  In1/1 -> Data Type Conversion10/1

== system gm_DUALportRAMinterface_v3_vnl/PL/integration_block1/Subsystem/a4_random ==
  In1 : Inport  OutDataTypeStr=uint16  PortDimensions=1  SampleTime=3.00000003e-08
  In2 : Inport  Port=2  OutDataTypeStr=boolean  PortDimensions=1  SampleTime=3.00000003e-08
  Add4 : Sum  Inputs=+-  OutDataTypeStr=fixdt(1, 18, 15)
  Add5 : Sum  OutDataTypeStr=fixdt(1, 17, 15)
  Bit Shift2 : hdlsllib/Logic and Bit Operations/Bit Shift  mode=Shift Right Logical  N=16+6
  Constant : Constant  OutDataTypeStr=boolean  SampleTime=Ts
  Constant2 : Constant  Value=-0.04  OutDataTypeStr=fixdt(1,18,15)  SampleTime=Ts
  Data Type Conversion6 : DataTypeConversion  OutDataTypeStr=fixdt(0,11,11)  SaturateOnIntegerOverflow=off  RndMeth=Floor
  Data Type Conversion7 : DataTypeConversion  OutDataTypeStr=fixdt(0,32,16)  SaturateOnIntegerOverflow=off  RndMeth=Floor
  Data Type Conversion8 : DataTypeConversion  OutDataTypeStr=fixdt(1,17,15)  SaturateOnIntegerOverflow=off  RndMeth=Floor
  Modulo by Constant HDL Optimized : embmathops/Modulo by Constant HDL Optimized  Denominator=0.008  SimulateUsing=Code generation
      settings: LibrarySourceBlock=|
      | embeddedMatrixLib/Math Operations/Modulo by Constant
      | HDL Optimized
  Switch2 : Switch  Criteria=u2 > Threshold  OutDataTypeStr=fixdt(1, 18, 15)  SaturateOnIntegerOverflow=off  InputSameDT=off
  mod_by_constant_term1 : Terminator
  Out1 : Outport  SampleTime=3.00000003e-08
  wires:
  Switch2/1 -> Out1/1
  Modulo by Constant HDL Optimized/2 -> mod_by_constant_term1/1
  Modulo by Constant HDL Optimized/1 -> Data Type Conversion8/1
  Data Type Conversion8/1 -> Add4/2, Add5/1
  Data Type Conversion7/1 -> Bit Shift2/1
  Data Type Conversion6/1 -> Modulo by Constant HDL Optimized/1
  Constant2/1 -> Add4/1, Add5/2
  Constant/1 -> Modulo by Constant HDL Optimized/2
  Bit Shift2/1 -> Data Type Conversion6/1
  Add5/1 -> Switch2/3
  Add4/1 -> Switch2/1
  In2/1 -> Switch2/2
  In1/1 -> Data Type Conversion7/1

== system gm_DUALportRAMinterface_v3_vnl/PL/integration_block1/Subsystem/b2_random ==
  In1 : Inport  OutDataTypeStr=uint16  PortDimensions=1  SampleTime=3.00000003e-08
  In2 : Inport  Port=2  OutDataTypeStr=boolean  PortDimensions=1  SampleTime=3.00000003e-08
  Add6 : Sum  Inputs=+-  OutDataTypeStr=fixdt(1, 18, 15)
  Add7 : Sum  OutDataTypeStr=fixdt(1, 18, 15)
  Bit Shift3 : hdlsllib/Logic and Bit Operations/Bit Shift  mode=Shift Right Logical  N=16+6
  Constant : Constant  OutDataTypeStr=boolean  SampleTime=Ts
  Constant3 : Constant  Value=-1.9970  OutDataTypeStr=fixdt(1,18,15)  SampleTime=Ts
  Data Type Conversion10 : DataTypeConversion  OutDataTypeStr=fixdt(0,32,16)  SaturateOnIntegerOverflow=off  RndMeth=Floor
  Data Type Conversion11 : DataTypeConversion  OutDataTypeStr=fixdt(1,18,15)  SaturateOnIntegerOverflow=off  RndMeth=Floor
  Data Type Conversion9 : DataTypeConversion  OutDataTypeStr=fixdt(0,11,11)  RndMeth=Floor
  Modulo by Constant HDL Optimized : embmathops/Modulo by Constant HDL Optimized  Denominator=0.0130  SimulateUsing=Code generation
      settings: LibrarySourceBlock=|
      | embeddedMatrixLib/Math Operations/Modulo by Constant
      | HDL Optimized
  Switch3 : Switch  Criteria=u2 > Threshold  OutDataTypeStr=fixdt(1, 18, 15)  SaturateOnIntegerOverflow=off  InputSameDT=off
  mod_by_constant_term1 : Terminator
  Out1 : Outport  SampleTime=3.00000003e-08
  wires:
  Switch3/1 -> Out1/1
  Modulo by Constant HDL Optimized/2 -> mod_by_constant_term1/1
  Modulo by Constant HDL Optimized/1 -> Data Type Conversion11/1
  Data Type Conversion9/1 -> Modulo by Constant HDL Optimized/1
  Data Type Conversion11/1 -> Add6/2, Add7/1
  Data Type Conversion10/1 -> Bit Shift3/1
  Constant3/1 -> Add6/1, Add7/2
  Constant/1 -> Modulo by Constant HDL Optimized/2
  Bit Shift3/1 -> Data Type Conversion9/1
  Add7/1 -> Switch3/3
  Add6/1 -> Switch3/1
  In2/1 -> Switch3/2
  In1/1 -> Data Type Conversion10/1

== system gm_DUALportRAMinterface_v3_vnl/PL/integration_block1/Subsystem/b3_random ==
  In1 : Inport  OutDataTypeStr=uint16  PortDimensions=1  SampleTime=3.00000003e-08
  In2 : Inport  Port=2  OutDataTypeStr=boolean  PortDimensions=1  SampleTime=3.00000003e-08
  Add6 : Sum  Inputs=+-  OutDataTypeStr=fixdt(1, 18, 15)
  Add7 : Sum  OutDataTypeStr=fixdt(1, 18, 15)
  Bit Shift3 : hdlsllib/Logic and Bit Operations/Bit Shift  mode=Shift Right Logical  N=16+6
  Constant : Constant  OutDataTypeStr=boolean  SampleTime=Ts
  Constant3 : Constant  Value=1.022  OutDataTypeStr=fixdt(1,18,15)  SampleTime=Ts
  Data Type Conversion10 : DataTypeConversion  OutDataTypeStr=fixdt(0,32,16)  SaturateOnIntegerOverflow=off  RndMeth=Floor
  Data Type Conversion11 : DataTypeConversion  OutDataTypeStr=fixdt(1,18,15)  SaturateOnIntegerOverflow=off  RndMeth=Floor
  Data Type Conversion9 : DataTypeConversion  OutDataTypeStr=fixdt(0,11,11)  RndMeth=Floor
  Modulo by Constant HDL Optimized : embmathops/Modulo by Constant HDL Optimized  Denominator=0.01  SimulateUsing=Code generation
      settings: LibrarySourceBlock=|
      | embeddedMatrixLib/Math Operations/Modulo by Constant
      | HDL Optimized
  Switch3 : Switch  Criteria=u2 > Threshold  OutDataTypeStr=fixdt(1, 18, 15)  SaturateOnIntegerOverflow=off  InputSameDT=off
  mod_by_constant_term1 : Terminator
  Out1 : Outport  SampleTime=3.00000003e-08
  wires:
  Switch3/1 -> Out1/1
  Modulo by Constant HDL Optimized/2 -> mod_by_constant_term1/1
  Modulo by Constant HDL Optimized/1 -> Data Type Conversion11/1
  Data Type Conversion9/1 -> Modulo by Constant HDL Optimized/1
  Data Type Conversion11/1 -> Add6/2, Add7/1
  Data Type Conversion10/1 -> Bit Shift3/1
  Constant3/1 -> Add6/1, Add7/2
  Constant/1 -> Modulo by Constant HDL Optimized/2
  Bit Shift3/1 -> Data Type Conversion9/1
  Add7/1 -> Switch3/3
  Add6/1 -> Switch3/1
  In2/1 -> Switch3/2
  In1/1 -> Data Type Conversion10/1

== system gm_DUALportRAMinterface_v3_vnl/PL/integration_block1/Subsystem/b4_random ==
  In1 : Inport  OutDataTypeStr=uint16  PortDimensions=1  SampleTime=3.00000003e-08
  In2 : Inport  Port=2  OutDataTypeStr=boolean  PortDimensions=1  SampleTime=3.00000003e-08
  Add8 : Sum  Inputs=+-  OutDataTypeStr=fixdt(1, 18, 15)
  Add9 : Sum  OutDataTypeStr=fixdt(1, 18, 16)
  Bit Shift4 : hdlsllib/Logic and Bit Operations/Bit Shift  mode=Shift Right Logical  N=16+12
  Constant : Constant  OutDataTypeStr=boolean  SampleTime=Ts
  Constant4 : Constant  Value=-0.0239  OutDataTypeStr=fixdt(1,18,15)  SampleTime=Ts
  Data Type Conversion12 : DataTypeConversion  OutDataTypeStr=fixdt(0,32,16)  SaturateOnIntegerOverflow=off  RndMeth=Floor
  Data Type Conversion13 : DataTypeConversion  OutDataTypeStr=fixdt(1,18,16)  SaturateOnIntegerOverflow=off  RndMeth=Floor
  Data Type Conversion14 : DataTypeConversion  OutDataTypeStr=fixdt(0,11,11)  SaturateOnIntegerOverflow=off  RndMeth=Floor
  Modulo by Constant HDL Optimized : embmathops/Modulo by Constant HDL Optimized  Denominator=2.5e-4  SimulateUsing=Code generation
      settings: LibrarySourceBlock=|
      | embeddedMatrixLib/Math Operations/Modulo by Constant
      | HDL Optimized
  Switch4 : Switch  Criteria=u2 > Threshold  OutDataTypeStr=fixdt(1, 18, 15)  SaturateOnIntegerOverflow=off  InputSameDT=off
  mod_by_constant_term1 : Terminator
  Out1 : Outport  SampleTime=3.00000003e-08
  wires:
  Switch4/1 -> Out1/1
  Modulo by Constant HDL Optimized/2 -> mod_by_constant_term1/1
  Modulo by Constant HDL Optimized/1 -> Data Type Conversion13/1
  Data Type Conversion14/1 -> Modulo by Constant HDL Optimized/1
  Data Type Conversion13/1 -> Add8/2, Add9/1
  Data Type Conversion12/1 -> Bit Shift4/1
  Constant4/1 -> Add8/1, Add9/2
  Constant/1 -> Modulo by Constant HDL Optimized/2
  Bit Shift4/1 -> Data Type Conversion14/1
  Add9/1 -> Switch4/3
  Add8/1 -> Switch4/1
  In2/1 -> Switch4/2
  In1/1 -> Data Type Conversion12/1

== system gm_DUALportRAMinterface_v3_vnl/PL/integration_block1/Subsystem/random_gene ==
  u1 : Inport  OutDataTypeStr=boolean  PortDimensions=1  SampleTime=3.00000003e-08
  u2 : Inport  Port=2  OutDataTypeStr=boolean  PortDimensions=1  SampleTime=3.00000003e-08
  In3 : Inport  Port=3  OutDataTypeStr=boolean  PortDimensions=1  SampleTime=3.00000003e-08
  In4 : Inport  Port=4  OutDataTypeStr=boolean  PortDimensions=1  SampleTime=3.00000003e-08
  Add12 : Sum  Inputs=++++  OutDataTypeStr=fixdt(0, 3, 0)
  Constant7 : Constant  OutDataTypeStr=fixdt(0,3,0)  SampleTime=Ts
  Data Type Conversion17 : DataTypeConversion  OutDataTypeStr=fixdt(0,3,0)  SaturateOnIntegerOverflow=off  RndMeth=Floor
  Data Type Conversion18 : DataTypeConversion  OutDataTypeStr=fixdt(0,3,0)  SaturateOnIntegerOverflow=off  RndMeth=Floor
  Data Type Conversion19 : DataTypeConversion  OutDataTypeStr=fixdt(0,3,0)  SaturateOnIntegerOverflow=off  RndMeth=Floor
  concat3 : hdlsllib/Logic and Bit Operations/Bit Concat  numInputs=2
  Out1 : Outport  SampleTime=3.00000003e-08
  wires:
  concat3/1 -> Data Type Conversion17/1
  Data Type Conversion19/1 -> Add12/1
  Data Type Conversion18/1 -> Add12/2
  Data Type Conversion17/1 -> Add12/4
  Constant7/1 -> Add12/3
  Add12/1 -> Out1/1
  In4/1 -> Data Type Conversion19/1
  In3/1 -> Data Type Conversion18/1
  u2/1 -> concat3/2
  u1/1 -> concat3/1

== system gm_DUALportRAMinterface_v3_vnl/PL/integration_block1/Subsystem/random_method ==
  u1 : Inport  OutDataTypeStr=boolean  PortDimensions=1  SampleTime=3.00000003e-08
  u2 : Inport  Port=2  OutDataTypeStr=boolean  PortDimensions=1  SampleTime=3.00000003e-08
  Add11 : Sum  OutDataTypeStr=fixdt(0, 3, 0)
  Constant6 : Constant  OutDataTypeStr=fixdt(0,3,0)  SampleTime=Ts
  Data Type Conversion16 : DataTypeConversion  OutDataTypeStr=fixdt(0,3,0)  SaturateOnIntegerOverflow=off  RndMeth=Floor
  concat2 : hdlsllib/Logic and Bit Operations/Bit Concat  numInputs=2
  Out1 : Outport  SampleTime=3.00000003e-08
  wires:
  concat2/1 -> Data Type Conversion16/1
  Data Type Conversion16/1 -> Add11/1
  Constant6/1 -> Add11/2
  Add11/1 -> Out1/1
  u2/1 -> concat2/2
  u1/1 -> concat2/1

== system gm_DUALportRAMinterface_v3_vnl/PL/integration_block1/Subsystem/random_sample ==
  u1 : Inport  OutDataTypeStr=boolean  PortDimensions=1  SampleTime=3.00000003e-08
  u2 : Inport  Port=2  OutDataTypeStr=boolean  PortDimensions=1  SampleTime=3.00000003e-08
  Add10 : Sum  OutDataTypeStr=fixdt(0, 4, 0)
  Constant5 : Constant  OutDataTypeStr=fixdt(0,4,0)  SampleTime=Ts
  Data Type Conversion15 : DataTypeConversion  OutDataTypeStr=fixdt(0,4,0)  SaturateOnIntegerOverflow=off  RndMeth=Floor
  concat1 : hdlsllib/Logic and Bit Operations/Bit Concat  numInputs=2
  Out1 : Outport  SampleTime=3.00000003e-08
  wires:
  concat1/1 -> Data Type Conversion15/1
  Data Type Conversion15/1 -> Add10/1
  Constant5/1 -> Add10/2
  Add10/1 -> Out1/1
  u2/1 -> concat1/2
  u1/1 -> concat1/1
